simulink model "imctmplni2bis"  (R2014a)
settings: Solver=ode45  StartTime=0.0  StopTime=1000000  RelTol=1e-3
undefined symbols (not defined in the file or in its folder): analoginput, analogoutput
libraries: daqlib x3, simulink x1
settings Model: ExtModeTrigMode=oneshot  ExtModeArmWhenConnect=off  Creator=auto2  LastModifiedBy=auto2
settings DataIOCC: LimitDataPoints=off  SignalLoggingSaveFormat=ModelDataLogs  SaveOutput=off  SaveTime=off  SignalLoggingName=sigsOut
settings OptimizationCC: BooleanDataType=off  ExpressionDepthLimit=2147483647  InitFltsAndDblsToZero=on
settings DebuggingCC: SaveWithParameterizedLinksMsg=none  UnderspecifiedInitializationDetection=Classic  SignalResolutionControl=TryResolveAllWithWarning  SolverPrmCheckMsg=none  MultiTaskDSMMsg=warning  MultiTaskCondExecSysMsg=none  FcnCallInpInsideContextMsg=UseLocalSettings  StateNameClashWarn=warning
settings HardwareCC: TargetUnknown=on
settings RTWCC: IncludeERTFirstTime=on
settings GRTTargetCC: CombineOutputUpdateFcns=off  GRTInterface=on

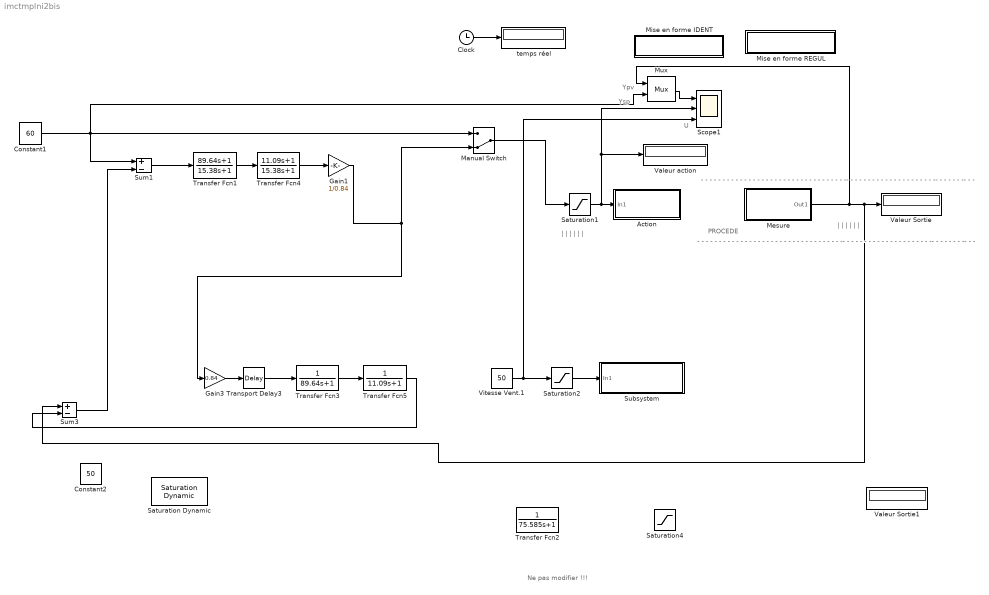
== system imctmplni2bis ==
  note: - - - - - - - - - - - - - - - - - - - - - - - - - - - - - - - - - -- - - - - - - - - - - - - - - - - - - - -- - - - - - - -- - -
  note: |
      | |
      | |
      | |
      | |
      | |
  note: |
      | |
      | |
      | |
      | |
      | |
  note: PROCEDE
  note: - - - - - - - - - - - - - - - - - - - - - - - - - - - - - - - - - -- - - - - - - - - - - - - - - - - - - - -- - - - - - -- - -
  note: Ypv
  note: Ysp
  note: U
  note: Ne pas modifier !!!
  Action : Subsystem
      mask Display: disp('Action \nPuissance')
  Clock : Clock
  Constant1 : Constant  Value=60
  Constant2 : Constant  Value=50
  Gain1 : Gain  Gain=1/0.84
  Gain3 : Gain  Gain=0.84
  Manual Switch : ManualSwitch  CurrentSetting=0
  Mesure : Subsystem
      mask Display: disp(' Mesure \n Température')
  Mise en forme IDENT : Subsystem
      settings: OpenFcn=t=ScopeData.time;A=[ScopeData.signals.values];y=A(:,1);u=A(:,3);plot(t,y,'black',t,u,'black');grid;figure(gcf)
      mask Display: disp('Mise en forme IDENT')
  Mise en forme REGUL : Subsystem
      settings: OpenFcn=|
      | t=ScopeData.time;
      | A=[ScopeData.signals.values];
      | y=A(:,1);
      | ysp=A(:,2);
      | u=A(:,3);
      | figure;
      | subplot(211);
      | plot(t,y,'black',t,ysp,'black');
      | grid;
      | title('Y_P_V - Y_S_P');
      | subplot(212),
      | plot(t,u,'black');
      | grid;
      | figure(gcf);
      | title('U')
      mask Display: disp('Mise en forme REGUL');
  Mux : Mux  Inputs=2
  Saturation Dynamic : simulink/Discontinuities/Saturation Dynamic  OutMin=[]  OutMax=[]  OutDataTypeStr=Inherit: Same as second input  OutDataType=fixdt(1, 16)  OutScaling=2^-10  DoSatur=off
  Saturation1 : Saturate  UpperLimit=100  LowerLimit=0
  Saturation2 : Saturate  UpperLimit=100  LowerLimit=0
  Saturation4 : Saturate  UpperLimit=100  LowerLimit=0
  Scope1 : Scope  NumInputPorts=3
      settings: TickLabels=on  TimeRange=800  YMin=35~0~0  YMax=65~100~100  MaxDataPoints=25000  SampleInput=on  SampleTime=1
  Subsystem : Subsystem
      mask Display: disp('commande en vitesse');
  Sum1 : Sum  Inputs=+-  SaturateOnIntegerOverflow=on
  Sum3 : Sum  Inputs=+-  SaturateOnIntegerOverflow=on
  Transfer Fcn1 : TransferFcn  Numerator=[89.64 1]  Denominator=[15.38 1]
  Transfer Fcn2 : TransferFcn  Denominator=[75.585 1]
  Transfer Fcn3 : TransferFcn  Numerator=1  Denominator=[89.64 1]
  Transfer Fcn4 : TransferFcn  Numerator=[11.09 1]  Denominator=[15.38 1]
  Transfer Fcn5 : TransferFcn  Numerator=1  Denominator=[11.09 1]
  Transport Delay3 : TransportDelay  DelayTime=13.84
  Valeur Sortie : Display
  Valeur Sortie1 : Display
  Valeur action : Display
  Vitesse Vent.1 : Constant  Value=50
  temps réel : Display
  wires:
  Mux/1 -> Scope1/1
  Saturation1/1 -> Scope1/2, Valeur action/1, Action/1(In1)
  Mesure/1(Out1) -> Sum3/1, Valeur Sortie/1, Mux/1
  Vitesse Vent.1/1 -> Saturation2/1, Scope1/3
  Saturation2/1 -> Subsystem/1(In1)
  Clock/1 -> temps réel/1
  Sum3/1 -> Sum1/2
  Sum1/1 -> Transfer Fcn1/1
  Transfer Fcn1/1 -> Transfer Fcn4/1
  Transfer Fcn4/1 -> Gain1/1
  Gain1/1 -> Gain3/1, Manual Switch/2
  Gain3/1 -> Transport Delay3/1
  Transport Delay3/1 -> Transfer Fcn3/1
  Transfer Fcn3/1 -> Transfer Fcn5/1
  Transfer Fcn5/1 -> Sum3/2
  Manual Switch/1 -> Saturation1/1
  Constant1/1 -> Mux/2, Manual Switch/1, Sum1/1

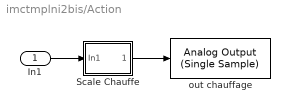
== system imctmplni2bis/Action ==
  In1 : Inport
  Scale Chauffe : Subsystem  mask(Mise à l'echelle){El=0, Eh=100, Il=2, Ih=10}
      mask prompts: El "Valeur basse du signal en entrée"; Eh "Valeur haute du signal en entrée"; Il "Valeur basse du signal en sortie"; Ih "Valeur haute du signal en sortie"
  out chauffage : daqlib/Analog Output (Single Sample)  DeviceMenu=nidaq Dev1 (PCI-6221 (37-pin))  Device=nidaq Dev1 (PCI-6221 (37-pin))  ObjConstructor=analogoutput('nidaq','Dev1')  NChannelsSelected=1  Channels=1$0$$1$0$#0$1$$1$0$#  NPorts=1 per hardware channel
  wires:
  Scale Chauffe/1(Out1) -> out chauffage/1
  In1/1 -> Scale Chauffe/1(In1)

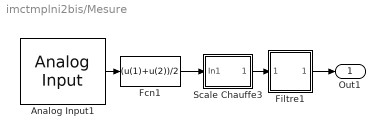
== system imctmplni2bis/Mesure ==
  Analog Input1 : daqlib/Analog Input  AcqMode=0  DeviceMenu=nidaq Dev1 (PCI-6221 (37-pin))  Device=nidaq Dev1 (PCI-6221 (37-pin))  ObjConstructor=analoginput('nidaq','Dev1')  SampleRate=10  ActualRate=10  SamplesPerFrame=2  InputType=SingleEnded  NChannelsSelected=1  Channels=1$0$$1$#0$1$$1$#0$2$$1$#0$3$$1$#0$4$$1$#0$5$$1$#0$6$$1$#0$7$$1$#0$8$$1$#0$9$$1$#0$10$$1$#0$11$$1$#0$12$$1$#0$13$$1$#0$14$$1$#0$15$$1$#  NPorts=1 per hardware channel  DataType=double
      settings: SignalType=Sample-based
  Fcn1 : Fcn  Expr=(u(1)+u(2))/2
  Filtre1 : Subsystem  mask(T){T=1}
      mask prompts: T "Constante de temps du filtre:"
  Scale Chauffe3 : Subsystem  mask(Mise à l'echelle){El=2, Eh=10, Il=0, Ih=100}
      mask prompts: El "Valeur basse du signal en entrée"; Eh "Valeur haute du signal en entrée"; Il "Valeur basse du signal en sortie"; Ih "Valeur haute du signal en sortie"
  Out1 : Outport
  wires:
  Analog Input1/1 -> Fcn1/1
  Fcn1/1 -> Scale Chauffe3/1(In1)
  Scale Chauffe3/1(Out1) -> Filtre1/1(In1)
  Filtre1/1(Out1) -> Out1/1

== system imctmplni2bis/Mise en forme IDENT ==

== system imctmplni2bis/Mise en forme REGUL ==

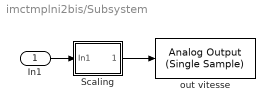
== system imctmplni2bis/Subsystem ==
  In1 : Inport
  Scaling : Subsystem  mask(Mise à l'echelle){El=0, Eh=100, Il=2, Ih=10}
      mask prompts: El "Valeur basse du signal en entrée"; Eh "Valeur haute du signal en entrée"; Il "Valeur basse du signal en sortie"; Ih "Valeur haute du signal en sortie"
  out vitesse : daqlib/Analog Output (Single Sample)  DeviceMenu=nidaq Dev1 (PCI-6221 (37-pin))  Device=nidaq Dev1 (PCI-6221 (37-pin))  ObjConstructor=analogoutput('nidaq','Dev1')  NChannelsSelected=1  Channels=0$0$$1$0$#1$1$$1$0$#  NPorts=1 per hardware channel
  wires:
  Scaling/1(Out1) -> out vitesse/1
  In1/1 -> Scaling/1(In1)

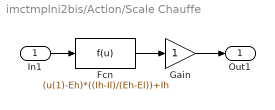
== system imctmplni2bis/Action/Scale Chauffe ==
  In1 : Inport
  Fcn : Fcn  Expr=(u(1)-Eh)*((Ih-Il)/(Eh-El))+Ih
  Gain : Gain  SampleTime=0.1  SaturateOnIntegerOverflow=on  OutDataTypeStr=Inherit: Same as input  ParamDataTypeStr=Inherit: Same as input
  Out1 : Outport
  wires:
  In1/1 -> Fcn/1
  Fcn/1 -> Gain/1
  Gain/1 -> Out1/1

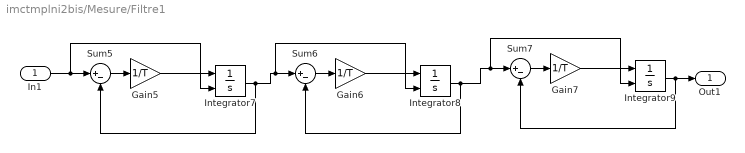
== system imctmplni2bis/Mesure/Filtre1 ==
  In1 : Inport
  Gain5 : Gain  Gain=1/T  SaturateOnIntegerOverflow=on  OutDataTypeStr=Inherit: Same as input  ParamDataTypeStr=Inherit: Same as input
  Gain6 : Gain  Gain=1/T  SaturateOnIntegerOverflow=on  OutDataTypeStr=Inherit: Same as input  ParamDataTypeStr=Inherit: Same as input
  Gain7 : Gain  Gain=1/T  SaturateOnIntegerOverflow=on  OutDataTypeStr=Inherit: Same as input  ParamDataTypeStr=Inherit: Same as input
  Integrator7 : Integrator  InitialConditionSource=external
  Integrator8 : Integrator  InitialConditionSource=external
  Integrator9 : Integrator  InitialConditionSource=external
  Sum5 : Sum  Inputs=|+-  SaturateOnIntegerOverflow=on  InputSameDT=on  OutDataTypeStr=Inherit: Same as first input
  Sum6 : Sum  Inputs=|+-  SaturateOnIntegerOverflow=on  InputSameDT=on  OutDataTypeStr=Inherit: Same as first input
  Sum7 : Sum  Inputs=|+-  SaturateOnIntegerOverflow=on  InputSameDT=on  OutDataTypeStr=Inherit: Same as first input
  Out1 : Outport
  wires:
  Sum5/1 -> Gain5/1
  Gain5/1 -> Integrator7/1
  In1/1 -> Sum5/1, Integrator7/2
  Sum6/1 -> Gain6/1
  Gain6/1 -> Integrator8/1
  Sum7/1 -> Gain7/1
  Gain7/1 -> Integrator9/1
  Integrator7/1 -> Sum5/2, Sum6/1, Integrator8/2
  Integrator8/1 -> Sum6/2, Sum7/1, Integrator9/2
  Integrator9/1 -> Sum7/2, Out1/1

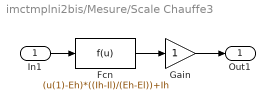
== system imctmplni2bis/Mesure/Scale Chauffe3 ==
  In1 : Inport
  Fcn : Fcn  Expr=(u(1)-Eh)*((Ih-Il)/(Eh-El))+Ih
  Gain : Gain  SampleTime=0.1  SaturateOnIntegerOverflow=on  OutDataTypeStr=Inherit: Same as input  ParamDataTypeStr=Inherit: Same as input
  Out1 : Outport
  wires:
  In1/1 -> Fcn/1
  Fcn/1 -> Gain/1
  Gain/1 -> Out1/1

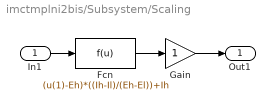
== system imctmplni2bis/Subsystem/Scaling ==
  In1 : Inport
  Fcn : Fcn  Expr=(u(1)-Eh)*((Ih-Il)/(Eh-El))+Ih
  Gain : Gain  SampleTime=0.1  SaturateOnIntegerOverflow=on  OutDataTypeStr=Inherit: Same as input  ParamDataTypeStr=Inherit: Same as input
  Out1 : Outport
  wires:
  Gain/1 -> Out1/1
  Fcn/1 -> Gain/1
  In1/1 -> Fcn/1
